simulink model "OLD_BIG_CCH_Model"  (R2023a)
settings: Solver=VariableStepAuto  StartTime=0.0  StopTime=10.0  RelTol=1e-3
values from neighbouring files (symbols this model uses):
  g = 9.80665    [coaxial_heli_parameters.m]    (also in initializeCCH.m)
  gamma_s = deg2rad(-0)    [coaxial_heli_parameters.m]    (also in initializeCCH.m = 0)
settings Model: Creator=prenc  LastModifiedBy=prenc

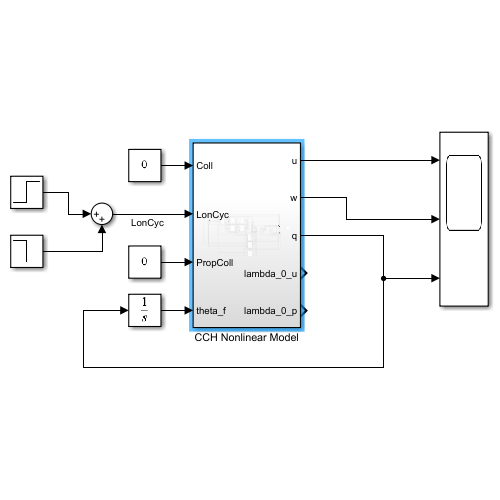
[thumbnail: Simulink's stored preview of the top-level diagram]
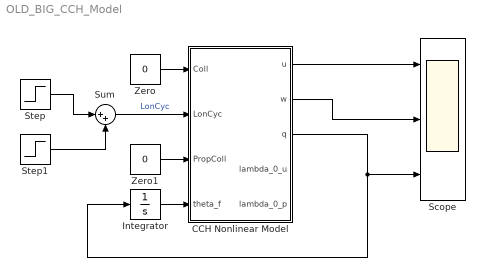
== system OLD_BIG_CCH_Model ==
  CCH Nonlinear Model : Subsystem
  Integrator : Integrator
  Scope : Scope  NumInputPorts=3
  Step : Step  SampleTime=0
  Step1 : Step  Time=2  After=-1  SampleTime=0
  Sum : Sum  Inputs=|++
  Zero : Constant  Value=0  OutDataTypeStr=Inherit: Inherit via back propagation
  Zero1 : Constant  Value=0  OutDataTypeStr=Inherit: Inherit via back propagation
  wires:
  Zero/1 -> CCH Nonlinear Model/1(Coll)
  Zero1/1 -> CCH Nonlinear Model/3(PropColl)
  CCH Nonlinear Model/3(q) -> Integrator/1, Scope/3
  Integrator/1 -> CCH Nonlinear Model/4(theta_f)
  Sum/1 -> CCH Nonlinear Model/2(LonCyc)  "LonCyc"
  Step/1 -> Sum/1
  Step1/1 -> Sum/2
  CCH Nonlinear Model/2(w) -> Scope/2
  CCH Nonlinear Model/1(u) -> Scope/1

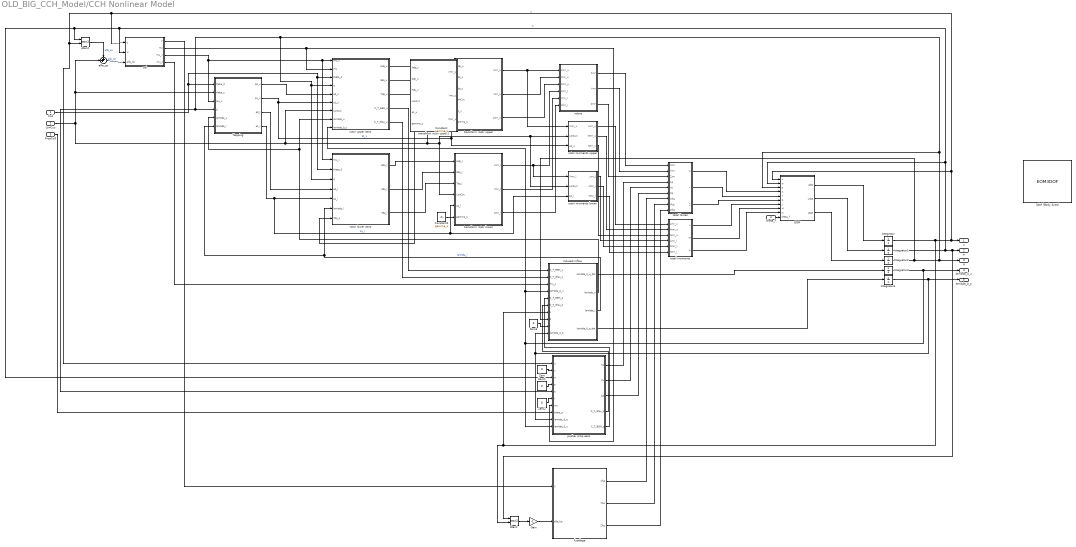
== system OLD_BIG_CCH_Model/CCH Nonlinear Model ==
  Coll : Inport
  LonCyc : Inport  Port=2
  PropColl : Inport  Port=3
  theta_f : Inport  Port=4
  3dof (Body Axes) : EOM3DOF  v_ini=0  mass=mass  Iyy=Iyy  g=g
  Atan1 : Trigonometry  Operator=atan2
  Atan2 : Trigonometry  Operator=atan2
  Constant : Constant  Value=gamma_s
  Constant1 : Constant  Value=gamma_s
  EOM : MATLAB Function  TreatAsAtomicUnit=on
  Gain : Gain  Gain=-1
  Integrator{,1..4} (5 alike) : Integrator
  Zero{,1..3} (4 alike) : Constant  Value=0  OutDataTypeStr=Inherit: Inherit via back propagation
  alfa_cp : Sum  Inputs=++|
  flapping : MATLAB Function  TreatAsAtomicUnit=on
  fuselage : MATLAB Function  TreatAsAtomicUnit=on
  induced inflow : MATLAB Function  TreatAsAtomicUnit=on
  pusher prop aero : MATLAB Function  TreatAsAtomicUnit=on
  rotor lower aero : MATLAB Function  TreatAsAtomicUnit=on
  rotor moments lower : MATLAB Function  TreatAsAtomicUnit=on
  rotor moments upper : MATLAB Function  TreatAsAtomicUnit=on
  rotor upper aero : MATLAB Function  TreatAsAtomicUnit=on
  rotors : MATLAB Function  TreatAsAtomicUnit=on
  total forces : MATLAB Function  TreatAsAtomicUnit=on
  total moments : MATLAB Function  TreatAsAtomicUnit=on
  transform rotor lower : MATLAB Function  TreatAsAtomicUnit=on
  transform rotor upper : MATLAB Function  TreatAsAtomicUnit=on
  transform rotor upper1 : MATLAB Function  TreatAsAtomicUnit=on
  vel : MATLAB Function  TreatAsAtomicUnit=on
  u : Outport
  w : Outport  Port=2
  q : Outport  Port=3
  lambda_0_u : Outport  Port=4
  lambda_0_p : Outport  Port=5
  wires:
  Coll/1 -> rotor lower aero/2(theta_0), rotor upper aero/3(theta_0), flapping/1(theta_0)
  Integrator/1 -> u/1, Atan2/2, pusher prop aero/1(u), vel/1(u), EOM/1(u), induced inflow/7(u), Atan1/2  "u"
  Integrator2/1 -> induced inflow/8(q), rotor lower aero/3(q), rotor upper aero/4(q), flapping/4(q), pusher prop aero/5(q), EOM/3(q), q/1
  Integrator3/1 -> lambda_0_u/1, rotor upper aero/9(lambda_0_u), induced inflow/4(lambda_0_u), pusher prop aero/10(lambda_0_u)
  alfa_cp/1 -> vel/3(alfa_cp)  "alfa_cp"
  Integrator1/1 -> Atan1/1, w/1, Atan2/1, pusher prop aero/3(w), vel/2(w), EOM/2(w)  "w"
  Atan2/1 -> alfa_cp/1  "alfa_sp"
  vel/3(mu_x) -> flapping/3(mu_x), rotor lower aero/1(mu_x), rotor upper aero/1(mu_x)
  Constant/1 -> transform rotor upper/6(gamma_s)
  flapping/1(a0_u) -> rotor upper aero/5(a0_u)
  flapping/2(a1_u) -> rotor moments upper/3(a1_u), transform rotor upper/5(a1_u), rotor upper aero/6(a1_u)  "a1_u"
  rotor upper aero/1(Hdp_u) -> transform rotor upper/1(Hdp_u)
  rotor upper aero/2(Sdp_u) -> transform rotor upper/2(Sdp_u)
  rotor upper aero/3(Tdp_u) -> transform rotor upper/3(Tdp_u), rotor lower aero/7(Tdp_u)
  rotor upper aero/4(C_T_BEM_u) -> induced inflow/1(C_T_BEM_u)
  rotor upper aero/5(C_T_Glau_u) -> induced inflow/2(C_T_Glau_u)
  vel/4(mu_z) -> induced inflow/3(mu_z)
  induced inflow/2(lambda_u) -> flapping/5(lambda_u), rotor upper aero/8(lambda_u)
  induced inflow/3(lambda_l) -> rotor lower aero/6(lambda_l), flapping/6(lambda_l)  "lambda_l"
  induced inflow/1(lambda_0_u_dot) -> Integrator3/1
  flapping/3(a0_l) -> rotor lower aero/4(a0_l)
  flapping/4(a1_l) -> rotor moments lower/3(a1_l), transform rotor lower/5(a1_l), rotor lower aero/5(a1_l)  "a1_l"
  rotor lower aero/1(Hdp_l) -> transform rotor lower/1(Hdp_l)
  rotor lower aero/2(Sdp_l) -> transform rotor lower/2(Sdp_l)
  rotor lower aero/3(Tdp_l) -> transform rotor lower/3(Tdp_l)
  Constant1/1 -> transform rotor lower/6(gamma_s)
  transform rotor upper/1(Xmr_u) -> rotor moments upper/1(Xmr_u), rotors/1(Xmr_u)
  transform rotor upper/2(Ymr_u) -> rotors/2(Ymr_u)
  transform rotor upper/3(Zmr_u) -> rotors/3(Zmr_u)
  transform rotor lower/1(Xmr_l) -> rotor moments lower/1(Xmr_l), rotors/4(Xmr_l)
  transform rotor lower/2(Ymr_l) -> rotors/5(Ymr_l)
  transform rotor lower/3(Zmr_l) -> rotors/6(Zmr_l)
  induced inflow/4(lambda_0_p_dot) -> Integrator4/1
  Zero/1 -> pusher prop aero/2(v)
  Zero1/1 -> pusher prop aero/4(p)
  Zero2/1 -> pusher prop aero/6(r)
  Integrator4/1 -> lambda_0_p/1, induced inflow/10(lambda_0_p), pusher prop aero/9(lambda_0_p)
  vel/2(mu) -> rotor upper aero/2(mu), pusher prop aero/7(mu)
  PropColl/1 -> pusher prop aero/8(theta_p)
  Atan1/1 -> Gain/1
  Gain/1 -> fuselage/2(alfa_fus)
  vel/1(V) -> fuselage/1(V)
  rotors/1(Xmr) -> total forces/1(Xmr)
  rotors/2(Ymr) -> total forces/2(Ymr)
  rotors/3(Zmr) -> total forces/3(Zmr)
  pusher prop aero/1(Xp) -> total forces/4(Xp)
  pusher prop aero/2(Yp) -> total forces/5(Yp)
  pusher prop aero/3(Zp) -> total forces/6(Zp)
  fuselage/1(Xfus) -> total forces/7(Xfus)
  fuselage/2(Yfus) -> total forces/8(Yfus)
  fuselage/3(Zfus) -> total forces/9(Zfus)
  total forces/3(Z) -> EOM/6(Z)
  total forces/1(X) -> EOM/4(X)
  total forces/2(Y) -> EOM/5(Y)
  EOM/1(udot) -> Integrator/1
  EOM/2(wdot) -> Integrator1/1
  EOM/3(qdot) -> Integrator2/1
  pusher prop aero/4(C_T_Glau_p) -> induced inflow/6(C_T_Glau_p)
  pusher prop aero/5(C_T_BEM_p) -> induced inflow/5(C_T_BEM_p)
  total moments/1(L) -> EOM/7(L)
  total moments/2(M) -> EOM/8(M)
  total moments/3(N) -> EOM/9(N)
  rotor moments lower/3(Nmr_l) -> total moments/6(Nmr_l)
  rotor moments lower/2(Mmr_l) -> total moments/5(Mmr_l)
  rotor moments lower/1(Lmr_l) -> total moments/4(Lmr_l)
  rotor moments upper/3(Nmr_u) -> total moments/3(Nmr_u)
  rotor moments upper/2(Mmr_u) -> total moments/2(Mmr_u)
  rotor moments upper/1(Lmr_u) -> total moments/1(Lmr_u)
  theta_f/1 -> EOM/10(theta_f)
  Zero3/1 -> induced inflow/9(r)
  LonCyc/1 -> transform rotor upper/4(LonCyc), rotor moments lower/2(LonCyc), rotor moments upper/2(LonCyc), transform rotor lower/4(LonCyc), rotor upper aero/7(LonCyc), alfa_cp/2, flapping/2(theta_c)

== matlab function OLD_BIG_CCH_Model/CCH Nonlinear Model/rotor lower aero ==
  data: mu_x input; Hdp_l output; theta_0 input; q input; a0_l input; a1_l input; lambda_l input; Tdp_u input; Sdp_l output; Tdp_l output
function [Hdp_l, Sdp_l, Tdp_l] = rotor_lower_aero(mu_x, theta_0, q, a0_l, a1_l, lambda_l, Tdp_u)
    
    c_l_a = rad2deg(0.1);
    Omega = 35;
    rho = 1.225;
    R = 5.49;
    sigma = 0.153;

    CHdp_l = sigma*0.015*mu_x/4 + sigma*c_l_a/4*((a1_l*mu_x^2/2 + mu_x*lambda_l)*theta_0/2 ...
        + q/Omega*(-a0_l/3) + (a0_l^2+a1_l^2)*mu_x/2);
    Hdp_l = CHdp_l * rho * (Omega*R)^2 * pi*R^2;

    Sdp_l = 0;

    Tdp_l = 2*Tdp_u;

end

== matlab function OLD_BIG_CCH_Model/CCH Nonlinear Model/transform rotor lower ==
  data: Hdp_l input; Sdp_l input; Tdp_l input; LonCyc input; a1_l input; Xmr_l output; gamma_s input; Ymr_l output; Zmr_l output
function [Xmr_l, Ymr_l, Zmr_l] = transform_rotor_lower(Hdp_l, Sdp_l, Tdp_l, LonCyc, a1_l, gamma_s)

    b1R_l = 0;
    gamma_s = deg2rad(-0);

    % Forces
    fmr_l_dp = [-Hdp_l; Sdp_l; -Tdp_l];

    a1R_l = LonCyc - a1_l;

    Tdp_b = [cos(a1R_l+gamma_s),    sin(a1R_l+gamma_s)*sin(b1R_l),  sin(a1R_l+gamma_s)*cos(b1R_l);
            0,                      cos(b1R_l),                     -sin(b1R_l);
            -sin(a1R_l+gamma_s),    cos(a1R_l+gamma_s)*sin(b1R_l),  cos(a1R_l+gamma_s)*cos(b1R_l)];

    fmr_l = Tdp_b * fmr_l_dp;

    Xmr_l = fmr_l(1); Ymr_l = fmr_l(2); Zmr_l = fmr_l(3);

    % Moments

end

== matlab function OLD_BIG_CCH_Model/CCH Nonlinear Model/rotors ==
  data: Xmr_u input; Xmr output; Ymr_u input; Zmr_u input; Xmr_l input; Ymr_l input; Zmr_l input; Ymr output; Zmr output
function [Xmr, Ymr, Zmr] = rotor(Xmr_u, Ymr_u, Zmr_u, Xmr_l, Ymr_l, Zmr_l)

    Xmr = Xmr_u + Xmr_l;
    Ymr = Ymr_u + Ymr_l;
    Zmr = Zmr_u + Zmr_l;

end

== matlab function OLD_BIG_CCH_Model/CCH Nonlinear Model/pusher prop aero ==
  data: u input; Xp output; Yp output; Zp output; v input; w input; p input; q input; r input; mu input; theta_p input; lambda_0_p input; C_T_Glau_p output; C_T_BEM_p output; lambda_0_u input
function [Xp, Yp, Zp, C_T_Glau_p, C_T_BEM_p] = pusher_propeller_aero(u, v, w, p, q, r, mu, theta_p, lambda_0_p, lambda_0_u)

    Kp = 0.4;
    Omega = 35;
    R = 5.49;
    l_p = 7.66;     % x location 
    h_p = 0;        % z location
    d_p = 0;        % y location
    omega_p = 207;
    R_p = 1.4;
    sigma_p = 0.142;
    c_l_a_p = 5.7;
    twist_p = deg2rad(-30);
    rho = 1.225;

    alfa_sp_p = atan2(w,u);
    mu_xp = sqrt(v^2 + (w + Kp*Omega*R*(lambda_0_u+2*lambda_0_u) + q*l_p)^2)/(omega_p*R_p);
    lambda_p = -(u-q*h_p-r*d_p)/(omega_p*R_p) - lambda_0_p;

    C_T_Glau_p = 2*lambda_0_p*sqrt( (mu*sin(alfa_sp_p))^2 + ...
        (mu*cos(alfa_sp_p)+lambda_0_p)^2 );       % this is like climbing flight for a rotor
    C_T_BEM_p = sigma_p*c_l_a_p/2*( (1/3+mu_xp^2/2)*theta_p + (1+mu_xp^2)/8*twist_p + lambda_p/2 );
    Tp = C_T_BEM_p * rho * (omega_p*R_p)^2 * pi*R_p^2;

    Xp = Tp; Yp = 0; Zp = 0;

end

== matlab function OLD_BIG_CCH_Model/CCH Nonlinear Model/rotor moments upper ==
  data: Xmr_u input; LonCyc input; Lmr_u output; Mmr_u output; Nmr_u output; a1_u input
function [Lmr_u, Mmr_u, Nmr_u] = rotor_moments_upper(Xmr_u, LonCyc, a1_u)
    
    Omega = 35;
    R = 5.49;
    hinge_offset_ratio = 0.05;
    m_bl = 50;
    gamma_s = deg2rad(-0);
    h_l = 0.89;                 % Shaft spacing upper rotor - Su et al. 2023   
    h_u = h_l + 0.77;

    Lmr_u = 0;
   
    a1r_u = LonCyc - a1_u;

    Me_u = (Omega*R)^2*hinge_offset_ratio*m_bl*sin(a1r_u+gamma_s);
    Mmr_u = -h_u*Xmr_u + Me_u; 

    Nmr_u = 0;

end

== matlab function OLD_BIG_CCH_Model/CCH Nonlinear Model/rotor moments lower ==
  data: Xmr_l input; LonCyc input; Lmr_l output; Mmr_l output; Nmr_l output; a1_l input
function [Lmr_l, Mmr_l, Nmr_l] = rotor_moments_lower(Xmr_l, LonCyc, a1_l)
    
    Omega = 35;
    R = 5.49;
    hinge_offset_ratio = 0.05;
    m_bl = 50;
    gamma_s = deg2rad(-0);
    h_l = 0.89;                 % Shaft spacing upper rotor - Su et al. 2023   

    Lmr_l = 0;

    a1r_l = LonCyc - a1_l;
    
    Me_l = (-Omega*R)^2*hinge_offset_ratio*m_bl*sin(a1r_l+gamma_s);
    Mmr_l = -h_l*Xmr_l + Me_l; 

    Nmr_l = 0;

end

== matlab function OLD_BIG_CCH_Model/CCH Nonlinear Model/fuselage ==
  data: V input; Xfus output; alfa_fus input; Yfus output; Zfus output
function [Xfus, Yfus, Zfus] = fuselage(V, alfa_fus)

    rho = 1.225;
    CDS = 1.9;

    Rfus = 0.5*rho*V^2*CDS*cos(alfa_fus);

    Xfus = -Rfus;
    Yfus = 0;
    Zfus = 0;

end

== matlab function OLD_BIG_CCH_Model/CCH Nonlinear Model/total forces ==
  data: Xmr input; X output; Ymr input; Zmr input; Xp input; Yp input; Zp input; Xfus input; Yfus input; Zfus input; Y output; Z output
function [X, Y, Z] = total_forces(Xmr, Ymr, Zmr, Xp, Yp, Zp, Xfus, Yfus, Zfus)

    X = Xmr + Xp + Xfus;
    Y = Ymr + Yp + Yfus;
    Z = Zmr + Zp + Zfus;

end

== matlab function OLD_BIG_CCH_Model/CCH Nonlinear Model/vel ==
  data: u input; V output; mu output; mu_x output; mu_z output; w input; alfa_cp input
function [V, mu, mu_x, mu_z] = vel(u, w, alfa_cp)

    Omega = 35;
    R = 5.49;

    V = sqrt(u^2+w^2);
    mu = V/(Omega*R);
    mu_x = V/(Omega*R) * cos(alfa_cp);
    mu_z = V/(Omega*R) * sin(alfa_cp);

end

== matlab function OLD_BIG_CCH_Model/CCH Nonlinear Model/total moments ==
  data: Lmr_u input; L output; Mmr_u input; Nmr_u input; M output; N output; Lmr_l input; Mmr_l input; Nmr_l input
function [L, M, N] = total_moments(Lmr_u, Mmr_u, Nmr_u, Lmr_l, Mmr_l, Nmr_l)

    L = Lmr_u + Lmr_l;
    M = Mmr_u + Mmr_l;
    N = Nmr_u + Nmr_l;

end

== matlab function OLD_BIG_CCH_Model/CCH Nonlinear Model/EOM ==
  data: u input; w input; q input; X input; Y input; Z input; udot output; wdot output; qdot output; L input; M input; N input; theta_f input
function [udot, wdot, qdot] = EOM(u,w, q, X, Y, Z, L, M ,N, theta_f)

    g = 9.80665;
    mass = 5500; 
    Iyy = 16000;

    udot = -q*w + X/mass -g*sin(theta_f);
    wdot = q*u + Z/mass + g*cos(theta_f);
    qdot = M/Iyy;

end

== matlab function OLD_BIG_CCH_Model/CCH Nonlinear Model/flapping ==
  data: a0_u output; a1_u output; a0_l output; a1_l output; theta_0 input; theta_c input; mu_x input; q input; lambda_u input; lambda_l input
function [a0_u, a1_u, a0_l, a1_l] = flapping(theta_0, theta_c, mu_x, q, lambda_u, lambda_l)
    
    hinge_offset_ratio = 0.05;
    nu_b2 = 1 + 3/2*hinge_offset_ratio/(1-hinge_offset_ratio);
    twist_r = deg2rad(-10);
    Omega = 35;
    lock = 6.57;

    a0_u = lock/(8*nu_b2) * (theta_0/2*(1+mu_x^2) + 4/3*lambda_u + twist_r*(4/5+2/3*mu_x) - 4/3*mu_x*theta_c);
    a0_l = lock/(8*nu_b2) * (theta_0/2*(1+mu_x^2) + 4/3*lambda_l + twist_r*(4/5+2/3*mu_x) - 4/3*mu_x*theta_c);
    a1_u = (8/3*mu_x*theta_0/2 + 2*mu_x*lambda_u - 16/lock*q/Omega + 2*twist_r*mu_x - (1+3/2*mu_x^2)*theta_c) / (1-1/2*mu_x^2); 
    a1_l = (8/3*mu_x*theta_0/2 + 2*mu_x*lambda_l - 16/lock*q/Omega + 2*twist_r*mu_x - (1+3/2*mu_x^2)*theta_c) / (1-1/2*mu_x^2); 


end

== matlab function OLD_BIG_CCH_Model/CCH Nonlinear Model/transform rotor upper1 ==
  data: Hdp_u input; Sdp_u input; Tdp_u input; LonCyc input; a1_u input; Xmr_u output; gamma_s input; Ymr_u output; Zmr_u output
function [Xmr_u, Ymr_u, Zmr_u] = transform_rotor_upper(Hdp_u, Sdp_u, Tdp_u, LonCyc, a1_u, gamma_s)

    b1R_u = 0;
    gamma_s = deg2rad(-0);

    a1R_u = LonCyc - a1_u;

    % Forces
    fmr_u_dp = [-Hdp_u; Sdp_u; -Tdp_u];

    Tdp_b = [cos(a1R_u+gamma_s),    sin(a1R_u+gamma_s)*sin(b1R_u),  sin(a1R_u+gamma_s)*cos(b1R_u);
            0,                      cos(b1R_u),                     -sin(b1R_u);
            -sin(a1R_u+gamma_s),    cos(a1R_u+gamma_s)*sin(b1R_u),  cos(a1R_u+gamma_s)*cos(b1R_u)];

    fmr_u = Tdp_b * fmr_u_dp;

    Xmr_u = fmr_u(1); Ymr_u = fmr_u(2); Zmr_u = fmr_u(3);

    % Moments

end

== matlab function OLD_BIG_CCH_Model/CCH Nonlinear Model/transform rotor upper ==
  data: Hdp_u input; Sdp_u input; Tdp_u input; LonCyc input; a1_u input; Xmr_u output; gamma_s input; Ymr_u output; Zmr_u output
function [Xmr_u, Ymr_u, Zmr_u] = transform_rotor_upper(Hdp_u, Sdp_u, Tdp_u, LonCyc, a1_u, gamma_s)

    b1R_u = 0;
    gamma_s = deg2rad(-0);

    a1R_u = LonCyc - a1_u;

    % Forces
    fmr_u_dp = [-Hdp_u; Sdp_u; -Tdp_u];

    Tdp_b = [cos(a1R_u+gamma_s),    sin(a1R_u+gamma_s)*sin(b1R_u),  sin(a1R_u+gamma_s)*cos(b1R_u);
            0,                      cos(b1R_u),                     -sin(b1R_u);
            -sin(a1R_u+gamma_s),    cos(a1R_u+gamma_s)*sin(b1R_u),  cos(a1R_u+gamma_s)*cos(b1R_u)];

    fmr_u = Tdp_b * fmr_u_dp;

    Xmr_u = fmr_u(1); Ymr_u = fmr_u(2); Zmr_u = fmr_u(3);

    % Moments

end

== matlab function OLD_BIG_CCH_Model/CCH Nonlinear Model/rotor upper aero ==
  data: mu_x input; mu input; Hdp_u output; theta_0 input; q input; a0_u input; a1_u input; LonCyc input; lambda_u input; lambda_0_u input; Sdp_u output; Tdp_u output; C_T_BEM_u output; C_T_Glau_u output
function [Hdp_u, Sdp_u, Tdp_u, C_T_BEM_u, C_T_Glau_u] = rotor_upper_aero(mu_x, mu, theta_0, q, a0_u, a1_u, LonCyc, lambda_u, lambda_0_u)
    
    c_l_a = rad2deg(0.1);
    Omega = 35;
    rho = 1.225;
    R = 5.49;
    sigma = 0.153;
    twist_r = deg2rad(-10);

    a1r_u = LonCyc - a1_u;

    CHdp_u = sigma*0.015*mu_x/4 + sigma*c_l_a/4*((a1_u*mu_x^2/2 + mu_x*lambda_u)*theta_0/2 ...
        + q/Omega*(-a0_u/3) + (a0_u^2+a1_u^2)*mu_x/2);
    Hdp_u = CHdp_u * rho * (Omega*R)^2 * pi*R^2;

    Sdp_u = 0;

    C_T_BEM_u = sigma*c_l_a/2*( (1/3+mu_x^2/2)*theta_0/2 + (1+mu_x^2)/8*twist_r + lambda_u/2 );
    C_T_Glau_u = 2*lambda_0_u * sqrt( (mu*cos(a1r_u))^2 + (mu*sin(a1r_u)+lambda_0_u)^2 );

    Tdp_u = C_T_BEM_u * rho * (Omega*R)^2 * pi*R^2;

end

== matlab function OLD_BIG_CCH_Model/CCH Nonlinear Model/induced inflow ==
  data: C_T_BEM_u input; lambda_0_u_dot output; C_T_Glau_u input; mu_z input; lambda_0_u input; lambda_u output; lambda_l output; C_T_BEM_p input; C_T_Glau_p input; lambda_0_p_dot output; u input; q input; r input; lambda_0_p input
function [lambda_0_u_dot, lambda_u, lambda_l, lambda_0_p_dot] = induced_inflow(C_T_BEM_u, C_T_Glau_u, mu_z, lambda_0_u, C_T_BEM_p, C_T_Glau_p, u, q, r, lambda_0_p)

    h_p = 0;     
    d_p = 0;     
    omega_p = 207;
    R_p = 1.4;

    % Main Rotors
    lambda_0_u_dot = (C_T_BEM_u-C_T_Glau_u)/0.1;
    lambda_u = (mu_z - lambda_0_u)/2;
    lambda_l = (mu_z - 2*lambda_0_u)/2;

    % Pusher Propeller
    lambda_0_p_dot = (C_T_BEM_p-C_T_Glau_p)/0.1;
    lambda_p = -(u-q*h_p-r*d_p)/(omega_p*R_p) - lambda_0_p;

end
